simulink model "ReglareaVitezeiMotorContinuu"  (R2023a)
settings: Solver=VariableStepAuto  StartTime=0.0  StopTime=0.05  RelTol=1e-3
values from neighbouring files (symbols this model uses):
  J = 5e-7    (= 5e-07)    [Date.m]
  k = 0.05    [Date.m]
  K_A = U / Uin    (= 2.4)    [Date.m]
  Ki = w^2/b    (= 1000)    [Date.m]
  Komg = Ui / (omg_max*Ktg)    (= 0.545415391248)    [Date.m]
  Kp = (2*tzeta*w - a) / b    (= 0.828)    [Date.m]
  Ktg = K_TG*60 / (2*pi*1000)    (= 0.0381971863421)    [Date.m]
  L = 1e-3    (= 0.001)    [Date.m]
  R = 10    [Date.m]
  Ue = 10    [Date.m]
settings Model: Creator=Bondrea  LastModifiedBy=Bondrea

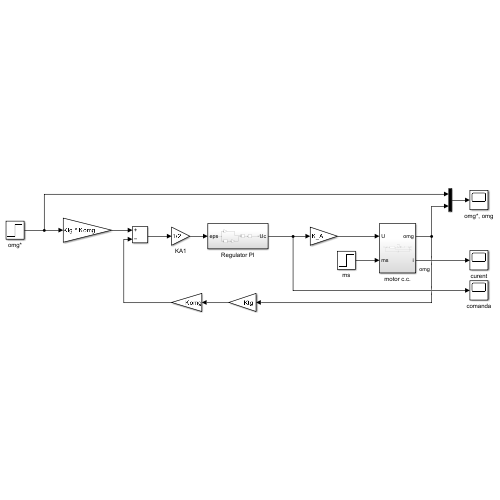
[thumbnail: Simulink's stored preview of the top-level diagram]
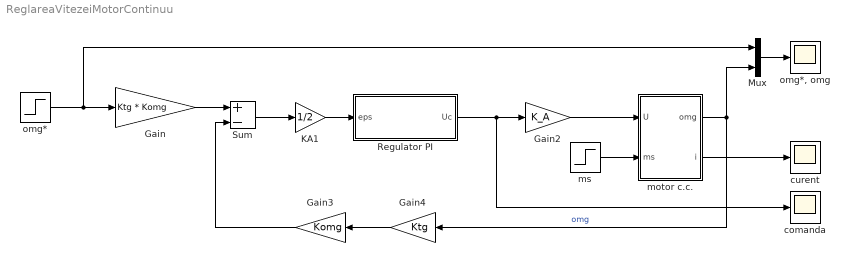
== system ReglareaVitezeiMotorContinuu ==
  Gain : Gain  Gain=Ktg * Komg
  Gain2 : Gain  Gain=K_A
  Gain3 : Gain  Gain=Komg
  Gain4 : Gain  Gain=Ktg
  KA1 : Gain  Gain=1/2
  Mux : Mux  Inputs=2
  Regulator PI : Subsystem
  Sum : Sum  Inputs=+-
  comanda : Scope
  curent : Scope
  motor c.c. : Subsystem
  ms : Step  Time=0.025  After=0.05  SampleTime=0
  omg* : Step  Before=240  After=240  SampleTime=0
  "omg*, omg" : Scope
  wires:
  KA1/1 -> Regulator PI/1(eps)
  Sum/1 -> KA1/1
  Gain/1 -> Sum/1
  Mux/1 -> "omg*, omg"/1
  Gain3/1 -> Sum/2
  Gain4/1 -> Gain3/1
  motor c.c./1(omg) -> Gain4/1, Mux/2  "omg"
  motor c.c./2(i) -> curent/1
  omg*/1 -> Mux/1, Gain/1
  Regulator PI/1(Uc) -> Gain2/1, comanda/1
  Gain2/1 -> motor c.c./1(U)
  ms/1 -> motor c.c./2(ms)

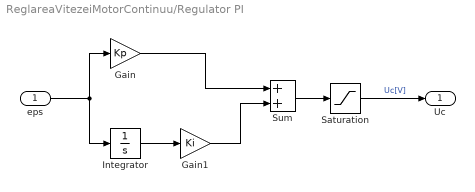
== system ReglareaVitezeiMotorContinuu/Regulator PI ==
  eps : Inport
  Gain : Gain  Gain=Kp
  Gain1 : Gain  Gain=Ki
  Integrator : Integrator
  Saturation : Saturate  UpperLimit=Ue  LowerLimit=-Ue
  Sum : Sum
  Uc : Outport
  wires:
  eps/1 -> Gain/1, Integrator/1
  Integrator/1 -> Gain1/1
  Gain1/1 -> Sum/2
  Gain/1 -> Sum/1
  Sum/1 -> Saturation/1
  Saturation/1 -> Uc/1  "Uc[V]"

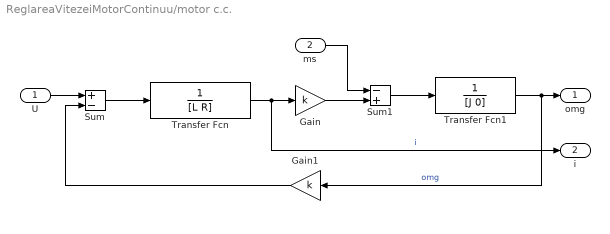
== system ReglareaVitezeiMotorContinuu/motor c.c. ==
  U : Inport
  ms : Inport  Port=2
  Gain : Gain  Gain=k
  Gain1 : Gain  Gain=k
  Sum : Sum  Inputs=+-
  Sum1 : Sum  Inputs=-+
  Transfer Fcn : TransferFcn  Denominator=[L R]
  Transfer Fcn1 : TransferFcn  Denominator=[J 0]
  omg : Outport
  i : Outport  Port=2
  wires:
  Sum/1 -> Transfer Fcn/1
  U/1 -> Sum/1
  Transfer Fcn/1 -> i/1, Gain/1  "i"
  Gain/1 -> Sum1/2
  ms/1 -> Sum1/1
  Sum1/1 -> Transfer Fcn1/1
  Transfer Fcn1/1 -> Gain1/1, omg/1  "omg"
  Gain1/1 -> Sum/2
